simulink model "Discretized_Linear_Controller_Linear_Plant_STATE_SPACE_Linear_Observer"  (R2025b)
settings: Solver=VariableStepAuto  StartTime=0.0  StopTime=10  RelTol=1e-3
values from neighbouring files (symbols this model uses):
  Aobs = [p.A_lin-L*C]    [drone_controller_with_observer.m]
  Bobs = [p.B_lin L]    [drone_controller_with_observer.m]
undefined symbols (not defined in the file or in its folder): DiscIntNeverNeededParam, K, p
libraries: discretizing x1
settings Model: Creator=chako  LastModifiedBy=chako

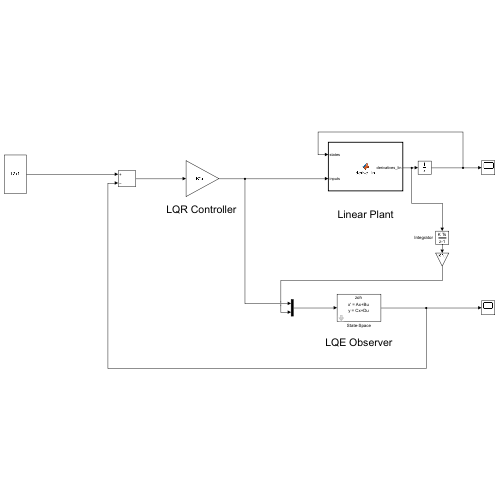
[thumbnail: Simulink's stored preview of the top-level diagram]
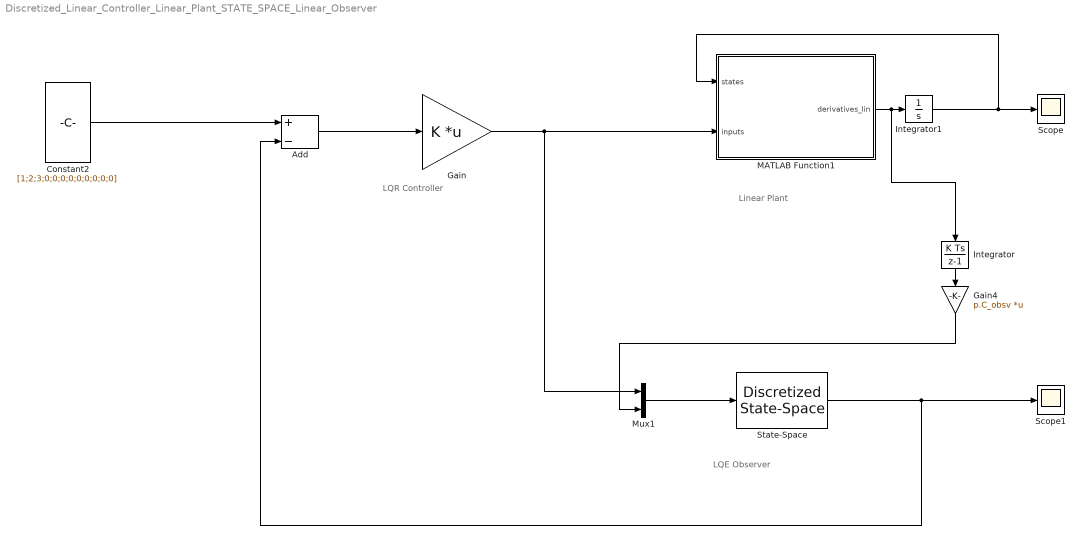
== system Discretized_Linear_Controller_Linear_Plant_STATE_SPACE_Linear_Observer ==
  note: Linear Plant
  note: LQR Controller
  note: LQE Observer
  Add : Sum  Inputs=+-
  Constant2 : Constant  Value=[1;2;3;0;0;0;0;0;0;0;0;0]
  Gain : Gain  Gain=K  Multiplication=Matrix(K*u)
  Gain4 : Gain  Gain=p.C_obsv  Multiplication=Matrix(K*u)
  Integrator : DiscreteIntegrator  SampleTime=0.0375  ICPrevOutput=DiscIntNeverNeededParam  ICPrevScaledInput=DiscIntNeverNeededParam  mask(DiscretizedDiscreteIntegrator){}
      mask init:
      | %zoh
  Integrator1 : Integrator
  MATLAB Function1 : MATLAB Function  TreatAsAtomicUnit=on
  Mux1 : Mux  Inputs=2
  Scope : Scope
      settings: ActiveDisplayYMinimum=-1.2083964498259996  ActiveDisplayYMaximum=4.653365768390449
  Scope1 : Scope
      settings: ActiveDisplayYMinimum=-2.5051596814278825  ActiveDisplayYMaximum=3.8302698641729163
  State-Space : discretizing/Discretized State-Space  A=Aobs  B=Bobs  C=eye(12)  D=zeros(12, 10)  ic=0  AbsTol=auto  SampleTime=0.0375  method=zoh  Wc=1
  wires:
  MATLAB Function1/1(derivatives_lin) -> Integrator1/1, Integrator/1
  Integrator/1 -> Gain4/1
  Constant2/1 -> Add/1
  Add/1 -> Gain/1
  Gain/1 -> MATLAB Function1/2(inputs), Mux1/1
  Gain4/1 -> Mux1/2
  State-Space/1 -> Add/2, Scope1/1
  Mux1/1 -> State-Space/1
  Integrator1/1 -> MATLAB Function1/1(states), Scope/1

== matlab function Discretized_Linear_Controller_Linear_Plant_STATE_SPACE_Linear_Observer/MATLAB Function1 ==
  data: states input size=12; derivatives_lin output size=12; inputs input size=4; p parameter
function derivatives_lin  = derive_lin(states, inputs, p)

    % Angles (roll, pitch, yaw) are small, approx 0
    % sin(x) = x, cos(x) = x 

    % Derivatives are zero
    % No torques (u2 to u4), but do need u1 = mg

    % eta is [phi, theta, psi] = roll pitch yaw
    xi= states(1:3); % x, y, z
    xid = states(4:6); %x_prime, y_prime, z_prime
    eta = states(7:9); % roll, pitch, yaw 
    etad = states(10:12); % roll_prime, pitch_prime, yaw_prime


    % Derivative of xi is xid

    % Calculative derivatives of xid
    % xidd = -(p.kD/p.m)*xid + [eta(2); -eta(1); 0]*p.g + [0;0;1]*inputs(1);
    % Calculative derivatives of etad
    % etadd = inputs
    A = [0 0 0   1 0 0           0 0 0   0 0 0;
         0 0 0   0 1 0           0 0 0   0 0 0;
         0 0 0   0 0 1           0 0 0   0 0 0;
         0 0 0   -p.kD/p.m 0 0   0 p.g 0   0 0 0;
         0 0 0   0 -p.kD/p.m 0   -p.g 0 0   0 0 0;
         0 0 0   0 0 -p.kD/p.m   0 0 0   0 0 0;
         0 0 0   0 0 0           0 0 0   1 0 0;
         0 0 0   0 0 0           0 0 0   0 1 0;
         0 0 0   0 0 0           0 0 0   0 0 1;
         0 0 0   0 0 0           0 0 0   0 0 0;
         0 0 0   0 0 0           0 0 0   0 0 0;
         0 0 0   0 0 0           0 0 0   0 0 0];

    B = [0 0 0 0;
         0 0 0 0;
         0 0 0 0;

         0 0 0 0;
         0 0 0 0;
         1/p.m 0 0 0;

         0 0 0 0;
         0 0 0 0;
         0 0 0 0;

         0 1/p.Ixx 0 0;
         0 0 1/p.Iyy 0;
         0 0 0 1/p.Izz;
         ];

    derivatives_lin = A * states + B * inputs;
end
